simulink model "pmsm_current_control"  (R2024b)
settings: Solver=VariableStepAuto  StartTime=0.0  StopTime=10.0  RelTol=1e-3
values from neighbouring files (symbols this model uses):
  Ki_id = 800.0    (= 800)    [simulate_surface_pmsm_foc.m]    (also in step2_build_current_loop_svpwm.m = 2 * pi * f_bw_id * Rs; step3_build_speed_loop.m = 2 * pi * f_bw_id * Rs; step4_build_position_loop.m = 2 * pi * 500 * Rs; step5b_current_control.m = 9424.77796077)
  Ki_iq = 800.0    (= 800)    [simulate_surface_pmsm_foc.m]    (also in step2_build_current_loop_svpwm.m = 2 * pi * f_bw_iq * Rs; step3_build_speed_loop.m = 2 * pi * f_bw_iq * Rs; step4_build_position_loop.m = 2 * pi * 500 * Rs; step5b_current_control.m = 9424.77796077)
  Kp_id = 40.0    (= 40)    [simulate_surface_pmsm_foc.m]    (also in step2_build_current_loop_svpwm.m = 2 * pi * f_bw_id * Ld_nom; step3_build_speed_loop.m = 2 * pi * f_bw_id * Ld_nom; step4_build_position_loop.m = 2 * pi * 500 * Ld_nom; step5b_current_control.m = 3.14159265359)
  Kp_iq = 40.0    (= 40)    [simulate_surface_pmsm_foc.m]    (also in step2_build_current_loop_svpwm.m = 2 * pi * f_bw_iq * Lq_nom; step3_build_speed_loop.m = 2 * pi * f_bw_iq * Lq_nom; step4_build_position_loop.m = 2 * pi * 500 * Lq_nom; step5b_current_control.m = 3.14159265359)
settings Model: Creator=Lee  LastModifiedBy=Lee

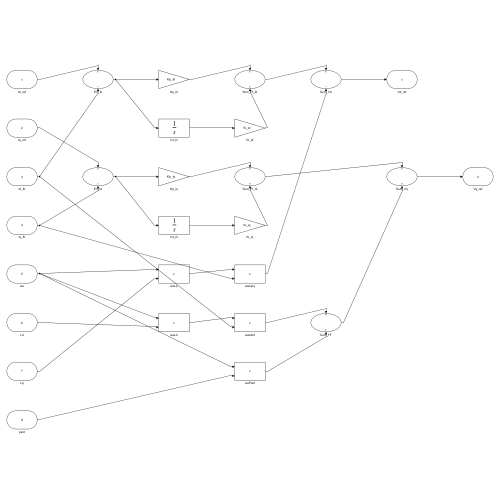
[thumbnail: Simulink's stored preview of the top-level diagram]
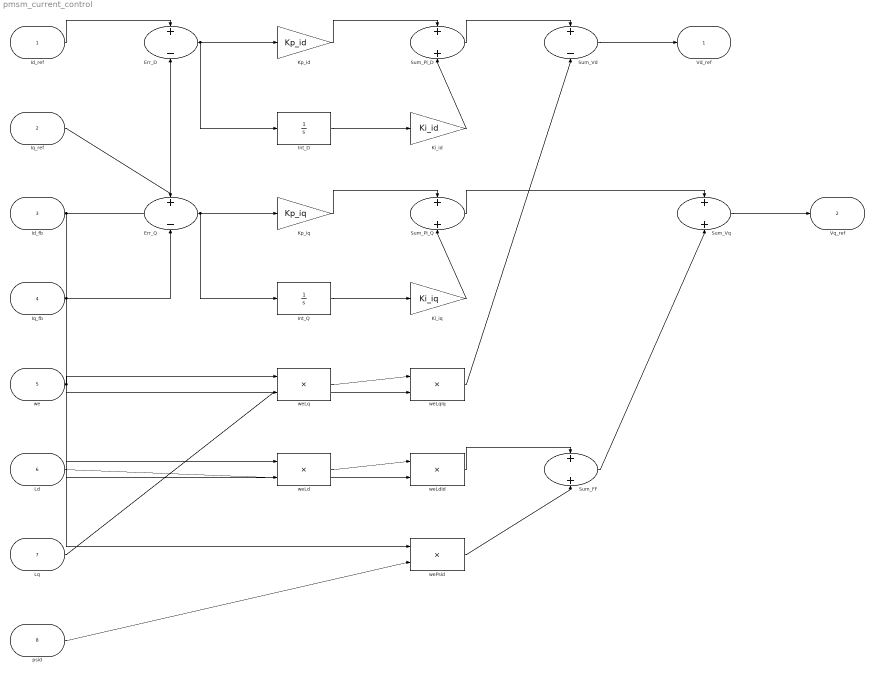
== system pmsm_current_control ==
  Id_ref : Inport
  Iq_ref : Inport  Port=2
  Id_fb : Inport  Port=3
  Iq_fb : Inport  Port=4
  we : Inport  Port=5
  Ld : Inport  Port=6
  Lq : Inport  Port=7
  psid : Inport  Port=8
  Err_D : Sum  Inputs=+-
  Err_Q : Sum  Inputs=+-
  Int_D : Integrator
  Int_Q : Integrator
  Ki_id : Gain  Gain=Ki_id
  Ki_iq : Gain  Gain=Ki_iq
  Kp_id : Gain  Gain=Kp_id
  Kp_iq : Gain  Gain=Kp_iq
  Sum_FF : Sum
  Sum_PI_D : Sum
  Sum_PI_Q : Sum
  Sum_Vd : Sum  Inputs=+-
  Sum_Vq : Sum
  weLd : Product
  weLdId : Product
  weLq : Product
  weLqIq : Product
  wePsid : Product
  Vd_ref : Outport
  Vq_ref : Outport  Port=2
  wires:
  Id_ref/1 -> Err_D/1
  Id_fb/1 -> Err_D/2, weLdId/2
  Err_D/1 -> Kp_id/1, Int_D/1
  Int_D/1 -> Ki_id/1
  Kp_id/1 -> Sum_PI_D/1
  Ki_id/1 -> Sum_PI_D/2
  we/1 -> weLq/1, weLd/1, wePsid/1
  Lq/1 -> weLq/2
  weLq/1 -> weLqIq/1
  Iq_fb/1 -> weLqIq/2, Err_Q/2
  Sum_PI_D/1 -> Sum_Vd/1
  weLqIq/1 -> Sum_Vd/2
  Sum_Vd/1 -> Vd_ref/1
  Iq_ref/1 -> Err_Q/1
  Err_Q/1 -> Kp_iq/1, Int_Q/1
  Int_Q/1 -> Ki_iq/1
  Kp_iq/1 -> Sum_PI_Q/1
  Ki_iq/1 -> Sum_PI_Q/2
  Ld/1 -> weLd/2
  weLd/1 -> weLdId/1
  psid/1 -> wePsid/2
  weLdId/1 -> Sum_FF/1
  wePsid/1 -> Sum_FF/2
  Sum_PI_Q/1 -> Sum_Vq/1
  Sum_FF/1 -> Sum_Vq/2
  Sum_Vq/1 -> Vq_ref/1
